simulink model "simu_MA"  (R2021a)
settings: Solver=VariableStepAuto  StartTime=0.0  StopTime=35944  RelTol=1e-3
values from neighbouring files (symbols this model uses):
  planta = tf(0.0001867, [1 0.0001919])    [ensaioMA.m]
  t_rp = []    [ensaioMA.m]
settings Model: Creator=jricl  LastModifiedBy=jricl

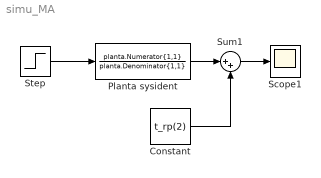
== system simu_MA ==
  Constant : Constant  Value=t_rp(2)
  Planta sysident : TransferFcn  Numerator=planta.Numerator{1,1}  Denominator=planta.Denominator{1,1}
  Scope1 : Scope
  Step : Step  Time=0  After=5  SampleTime=1
  Sum1 : Sum  Inputs=|++
  wires:
  Constant/1 -> Sum1/2
  Sum1/1 -> Scope1/1
  Planta sysident/1 -> Sum1/1
  Step/1 -> Planta sysident/1
